simulink library "Suspension_Systems"  (R2020a)
settings: Solver=VariableStepAuto  StartTime=0.0  StopTime=10.0  RelTol=1e-3
undefined symbols (not defined in the file): Init, Vehicle
libraries: Suspension_Linkage x1, Susp_LiveAxle x1, Susp_DOF15 x1
Description:
  | Component of Simscape Vehicle Templates Library
  | 
  | Copyright 2018-2021 The MathWorks, Inc.
settings Model: Creator=smiller  LastModifiedBy=smiller
settings DataIOCC: ReturnWorkspaceOutputs=off
settings DebuggingCC: ArithmeticOperatorsInVariantConditions=warning
settings SFSimCC: CustomCodeUndefinedFunction=UseInterfaceOnly

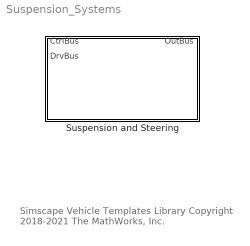
== system Suspension_Systems ==
  note: Simscape Vehicle Templates Library
      | Copyright 2018-2021 The MathWorks, Inc.
  Suspension and Steering : Subsystem  Variant=on  VariantControlMode=Label  VariantControl=Variant1  LabelModeActiveChoice=Simple  mask(Suspension and Steering){Susp=Vehicle.Chassis.SuspA1, Init=Init.Axle1, VariantLabel=Vehicle.Chassis.SuspA1.class.Value, InitTriggerDropdown=1}
      mask prompts: Susp "Suspension Parameters"; Init "Initial Values"; VariantLabel "Variant Label"; InitTriggerDropdown "Initialization Trigger Dropdown"
      mask init:
      | curblk = gcb;
      | 
      | % Set variant for this block 
      | set_param(curblk,'LabelModeActiveChoice',VariantLabel);
      | 
      | % Trigger Mask Initialization for 
      | % variant subsystems below this level
      | sm_car_lib_maskInitTrigger(curblk)
      mask TypeOptions InitTriggerDropdown: 0 | 1
      mask Display:
      | blk = find_system(gcbh, 'LookUnderMasks', 'all', 'SearchDepth', 1,'FollowLinks','on', 'Parent', gcb,'VariantObject', get_param(gcb,'activevariant'));
      | eval(get_param(blk, 'MaskDisplay'));

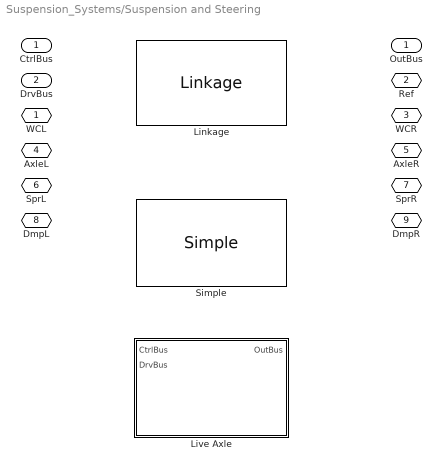
== system Suspension_Systems/Suspension and Steering ==
  "CtrlBus " : Inport
  DrvBus : Inport  Port=2
  Linkage : Suspension_Linkage/Linkage  VariantControl=Linkage  InitTriggerDropdown=1
  Live Axle : Subsystem  VariantControl=LiveAxle  mask(Live Axle){LiveAxle=Susp.LiveAxle}
      mask prompts: LiveAxle "Live Axle (structure)"
      mask help: Live Axle Suspension
      mask Display: image('sm_car_vehicle_susp_liveaxle_IMAGE.png');
  Simple : Susp_DOF15/Simple  VariantControl=Simple  InitTriggerDropdown=1
  WCL : PMIOPort  Side=Left
  Ref : PMIOPort  Port=2  Side=Right
  WCR : PMIOPort  Port=3  Side=Right
  AxleL : PMIOPort  Port=4  Side=Left
  AxleR : PMIOPort  Port=5  Side=Right
  SprL : PMIOPort  Port=6  Side=Left
  SprR : PMIOPort  Port=7  Side=Right
  DmpL : PMIOPort  Port=8  Side=Left
  DmpR : PMIOPort  Port=9  Side=Right
  OutBus : Outport  VectorParamsAs1DForOutWhenUnconnected=off

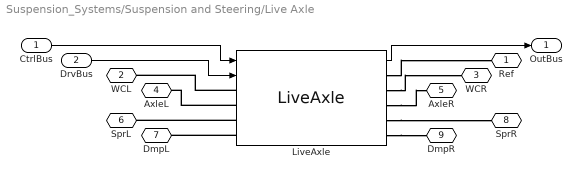
== system Suspension_Systems/Suspension and Steering/Live Axle ==
  CtrlBus : Inport
  DrvBus : Inport  Port=2
  LiveAxle : Susp_LiveAxle/LiveAxle  VariantControl=LiveAxle  Init=Init  hp_shock_top=LiveAxle.Shock.sTop.Value  hp_shock_bot=LiveAxle.Shock.sBottom.Value  hp_leaf_body=LiveAxle.Leaf.sBody.Value  hp_leaf_axle=LiveAxle.Leaf.sAxle.Value  hp_whl_ctr=LiveAxle.sWheelCentre.Value  axle_rad=LiveAxle.Axle.radius.Value  axle_mass=LiveAxle.Axle.m.Value  leaf_w=LiveAxle.Leaf.xWidth.Value  leaf_t=LiveAxle.Leaf.xThickness.Value  leaf_rho=LiveAxle.Leaf.density.Value  leaf_E=LiveAxle.Leaf.E.Value  leaf_nu=LiveAxle.Leaf.nu.Value  leaf_zeta=LiveAxle.Leaf.zDamping.Value  piston_mass=LiveAxle.Shock.mPiston.Value  cyl_mass=LiveAxle.Shock.mCylinder.Value  shock_xmax=LiveAxle.Endstop.xMax.Value  shock_xmin=LiveAxle.Endstop.xMin.Value
  Ref : PMIOPort  Side=Right
  WCL : PMIOPort  Port=2  Side=Left
  WCR : PMIOPort  Port=3  Side=Right
  AxleL : PMIOPort  Port=4  Side=Left
  AxleR : PMIOPort  Port=5  Side=Right
  SprL : PMIOPort  Port=6  Side=Left
  DmpL : PMIOPort  Port=7  Side=Left
  SprR : PMIOPort  Port=8  Side=Right
  DmpR : PMIOPort  Port=9  Side=Right
  OutBus : Outport  VectorParamsAs1DForOutWhenUnconnected=off
  wires:
  LiveAxle/1 -> OutBus/1
  CtrlBus/1 -> LiveAxle/1
  DrvBus/1 -> LiveAxle/2
  connections:
  LiveAxle/LConn4 -- DmpL/RConn1
  LiveAxle/LConn3 -- SprL/RConn1
  LiveAxle/RConn3 -- AxleR/RConn1
  LiveAxle/LConn2 -- AxleL/RConn1
  LiveAxle/LConn1 -- WCL/RConn1
  LiveAxle/RConn1 -- Ref/RConn1
  LiveAxle/RConn4 -- SprR/RConn1
  LiveAxle/RConn2 -- WCR/RConn1
  LiveAxle/RConn5 -- DmpR/RConn1
